simulink model "Copy_of_PDUSTM32"  (R2024b)
settings: Solver=FixedStepDiscrete  StartTime=0.0  StopTime=1  FixedStep=0.001  RelTol=1e-3  EnableMultiTasking=on
libraries: stm32blockslib x32, stm32f4xxblockslib x14, canmsglib x7, simulink x3, stm32h7xxblockslib x1
(part 1 of 3)
settings Model: STM32="{\"DigitalPortRead\":[{\"ID\":\"Copy_of_PDUSTM32:620\"},{\"ID\":\"Copy_of_PDUSTM32:1176\"},{\"ID\":\"Copy_of_PDUSTM32:1323\"}],\"SPIControllerTransfer\":[{\"ID\":\"Copy_of_PDUSTM32:1123\"},{\"ID\":\"Copy_of_PDUSTM32:1124\"},{\"ID\":\"Copy_of_PDUSTM32:1150\"},{\"ID\":\"Copy_of_PDUSTM32:1151\"},{\"ID\":\"Copy_of_PDUSTM32:1152\"},{\"ID\":\"Copy_of_PDUSTM32:1153\"},{\"ID\":\"Copy_of_PDUSTM32:1154\"},{\"ID\":\"Copy_of_PDUSTM32:1155\"},{\"ID\":\"Copy_of_PDUSTM32:1156\"},{\"ID\":\"Copy_of_PDUSTM32:1157\"},{\"ID\":\"Copy_of_PDUSTM32:709\"},{\"ID\":\"Copy_of_PDUSTM32:716\"},{\"ID\":\"Copy_of_PDUSTM32:722\"},{\"ID\":\"Copy_of_PDUSTM32:728\"},{\"ID\":\"Copy_of_PDUSTM32:1255\"},{\"ID\":\"Copy_of_PDUSTM32:1256\"},{\"ID\":\"Copy_of_PDUSTM32:1270\"},{\"ID\":\"Copy_of_PDUSTM32:1271\"},{\"ID\":\"Copy_of_PDUSTM32:1285\"},{\"ID\":\"Copy_of_PDUSTM32:1286\"},{\"ID\":\"Copy_of_PDUSTM32:1305\"},{\"ID\":\"Copy_of_PDUSTM32:1306\"},{\"ID\":\"Copy_of_PDUSTM32:1181\"},{\"ID\":\"Copy_of_PDUSTM32:1328\"},{\"ID\":\"Copy_of_PDUSTM32:1365\"},{\"ID\":\"Copy_of_PDUSTM32:1366\"},{\"ID\":\"Copy_of_PDUSTM32:1382\"},{\"ID\":\"Copy_of_PDUSTM32:1383\"},{\"ID\":\"Copy_of_PDUSTM32:1394\"},{\"ID\":\"Copy_of_PDUSTM32:1395\"},{\"ID\":\"Copy_of_PDUSTM32:1406\"},{\"ID\":\"Copy_of_PDUSTM32:1407\"}],\"AnalogInputForH7\":{\"ID\":\"Copy_of_PDUSTM32:731\"},\"DigitalPortWrite\":[{\"ID\":\"Copy_of_PDUSTM32:1095\"},{\"ID\":\"Copy_of_PDUSTM32:1094\"},{\"ID\":\"Copy_of_PDUSTM32:1093\"},{\"ID\":\"Copy_of_PDUSTM32:1092\"},{\"ID\":\"Copy_of_PDUSTM32:1091\"},{\"ID\":\"Copy_of_PDUSTM32:826\"},{\"ID\":\"Copy_of_PDUSTM32:825\"},{\"ID\":\"Copy_of_PDUSTM32:809\"},{\"ID\":\"Copy_of_PDUSTM32:921\"},{\"ID\":\"Copy_of_PDUSTM32:889\"},{\"ID\":\"Copy_of_PDUSTM32:1131\"}]}"  Creator=will  LastModifiedBy=Will
settings SolverCC: AlgebraicLoopSolver=TrustRegion
settings DataIOCC: ReturnWorkspaceOutputs=off
settings OptimizationCC: DefaultParameterBehavior=Inlined  EnhancedBackFolding=on  PassReuseOutputArgsAs=Individual arguments  ZeroExternalMemoryAtStartup=off  ZeroInternalMemoryAtStartup=off  MaxStackSize=512  OptimizeBlockOrder=speed  DifferentSizesBufferReuse=on  OptimizationCustomize=off  EfficientTunableParamExpr=on
settings DebuggingCC: ParameterTunabilityLossMsg=error  UnconnectedInputMsg=warning  UnconnectedOutputMsg=warning  UnconnectedLineMsg=warning  ArithmeticOperatorsInVariantConditions=warning
settings HardwareCC: ProdBitPerPointer=32  ProdBitPerSizeT=32  ProdBitPerPtrDiffT=32  ProdLargestAtomicInteger=Long  ProdLargestAtomicFloat=Double  ProdWordSize=32  ProdLongLongMode=on  ProdHWDeviceType=ARM Compatible->ARM Cortex-M
settings ModelReferenceCC: EnableRefExpFcnMdlSchedulingChecks=on
settings SFSimCC: MATLABDynamicMemAlloc=off  CustomCodeUndefinedFunction=UseInterfaceOnly
settings RTWCC: Description=Embedded Coder  SystemTargetFile=ert.tlc  HardwareBoard=STM32H7xx Based (Single-core)  TemplateMakefile=ert_default_tmf  CustomHeaderCode="#include \"stm32h7xx_ll_tim.h\""  CustomInitializer=LL_TIM_EnableCounter(TIM2);  Toolchain=GNU Tools for ARM Embedded Processors  GPUComputeCapability=3.5
settings CodeAppCC: ForceParamTrailComments=on  IgnoreCustomStorageClasses=off  OperatorAnnotations=on  SimulinkDataObjDesc=on  SFDataObjDesc=on  InsertBlockDesc=on
settings ERTTargetCC: TargetLangStandard=C99 (ISO)  CodeReplacementLibrary=ARM Cortex-M  ExtModeTransport=3  ExtModeStaticAlloc=on  ExtModeStaticAllocSize=2048  ExtModeMexFile=ext_xcp  ExtModeIntrfLevel=Level2 - Open

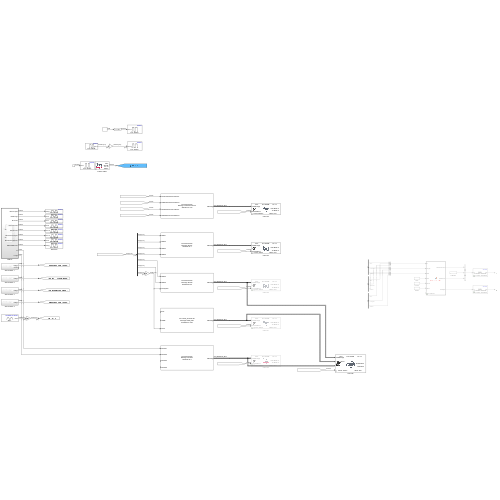
[thumbnail: Simulink's stored preview of the top-level diagram]
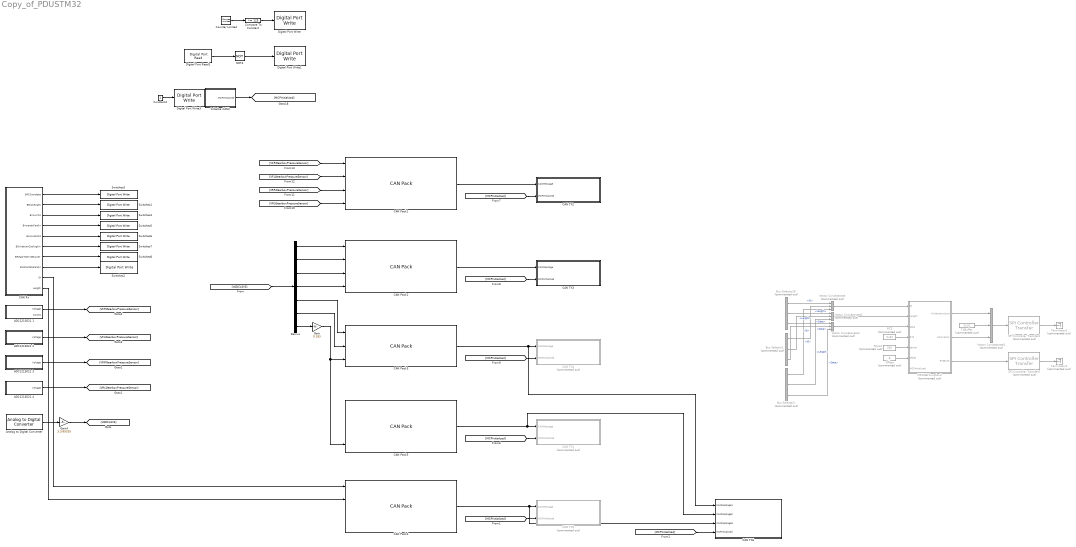
== system Copy_of_PDUSTM32 ==
  ADC121S021 1 : Subsystem
  ADC121S021 2 : Subsystem
  ADC121S021 3 : Subsystem
  ADC121S021 4 : Subsystem
  Analog to Digital Converter : stm32h7xxblockslib/Analog to Digital Converter  ADCModule=ADC1  ConversionGroup=Regular  TriggerMode=Read results only  NumberOfConversions=7  EnableBufferConv=off  BufferLength=1  OutputStatus=off  SampleTime=-1  EnableSimPort=off  hoistedMaskSrc=ECSoC/ECSimCodegen/Analog to Digital Converter
  Bus Selector1 : BusSelector  Commented=on  OutputSignals=ID,Length,Data
  Bus Selector16 : BusSelector  Commented=on  OutputSignals=ID,Length,Data
  Bus Selector2 : BusSelector  Commented=on  OutputSignals=ID,Length,Data
  CAN Pack1 : canmsglib/CAN Pack  CANdbFile=C:\Users\oxbro\Documents\STM32CustomProjects\PDUSTM32\ADCTest.dbc  MsgList=GearboxPressures  MsgName=GearboxPressures  MsgIDType=Standard (11-bit identifier)  MsgIdentifier=105  CANIDInput=off  MsgLength=8  Remote=off  ApplyMinMax=off  BusOutput=on  SignalInfo={'VFLGearboxPressureSensor','0','12','LE','unsigned','Standard','0','0.0012211','0','0','5.0004';'VFRGearboxPressureSensor','16','12','LE','unsigned','Standard','0','0.0012211','0','0','5.0004';'VRLGearboxPressureSensor','32','12','LE','unsigned','Standard','0','0.0012211','0','0','5.0004';'VRRGearboxPressureSensor','48','12','LE','unsigned','Standard','0','0.0012211','0','0','5.0004'}
      settings: LibrarySourceBlock=stmutilitieslib/CAN Pack  DataFormat=CANdb specified signals
  CAN Pack2 : canmsglib/CAN Pack  CANdbFile=C:\Users\oxbro\Documents\STM32CustomProjects\PDUSTM32\ADCTest.dbc  MsgList=ADCs1  MsgName=ADCs1  MsgIDType=Standard (11-bit identifier)  MsgIdentifier=5  CANIDInput=off  MsgLength=8  Remote=off  ApplyMinMax=off  BusOutput=on  SignalInfo={'VADC1','0','16','LE','unsigned','Standard','0','5.04e-05','0','0','3.303';'VADC2','16','16','LE','unsigned','Standard','0','5.04e-05','0','0','3.303';'VADC3','32','16','LE','unsigned','Standard','0','5.04e-05','0','0','3.303';'VADC4','48','16','LE','unsigned','Standard','0','5.04e-05','0','0','3.303'}
      settings: LibrarySourceBlock=stmutilitieslib/CAN Pack  DataFormat=CANdb specified signals
  CAN Pack3 : canmsglib/CAN Pack  CANdbFile=C:\Users\oxbro\Documents\STM32CustomProjects\PDUSTM32\ADCTest.dbc  MsgList=ADCs2  MsgName=ADCs2  MsgIDType=Standard (11-bit identifier)  MsgIdentifier=66  CANIDInput=off  MsgLength=6  Remote=off  ApplyMinMax=off  BusOutput=on  SignalInfo={'VADC5','0','16','LE','unsigned','Standard','0','5.04e-05','0','0','3.303';'VADC6','16','16','LE','unsigned','Standard','0','5.04e-05','0','0','3.303';'VLVSystem','32','16','LE','unsigned','Standard','0','0.00046327','0','0','30.3604'}
      settings: LibrarySourceBlock=stmutilitieslib/CAN Pack  DataFormat=CANdb specified signals
  CAN Pack4 : canmsglib/CAN Pack  CANdbFile=C:\Users\oxbro\Documents\STM32CustomProjects\PDUSTM32\ADCTest.dbc  MsgList=Numbers  MsgName=Numbers  MsgIDType=Standard (11-bit identifier)  MsgIdentifier=0  CANIDInput=off  MsgLength=8  Remote=off  ApplyMinMax=off  BusOutput=on  SignalInfo={'Number1','0','16','LE','signed','Standard','0','1','0','-32768','32767';'Number2','16','16','LE','signed','Standard','0','1','0','-32768','32767';'Number3','32','16','LE','signed','Standard','0','1','0','-32768','32767';'Number4','48','16','LE','signed','Standard','0','1','0','-32768','32767'}
      settings: LibrarySourceBlock=stmutilitieslib/CAN Pack  DataFormat=CANdb specified signals
  CAN Pack5 : canmsglib/CAN Pack  CANdbFile=C:\Users\Will\Desktop\OBR\Embedded\PDUSTM32\CAN3_28.06.26.dbc  MsgList=PDM_Data  MsgName=PDM_Data  MsgIDType=Standard (11-bit identifier)  MsgIdentifier=1328  CANIDInput=off  MsgLength=8  Remote=off  ApplyMinMax=off  BusOutput=on  SignalInfo={'ILVS','8','8','LE','unsigned','Standard','0','1','0','0','255';'TPDM','16','8','LE','unsigned','Standard','0','1','0','0','255';'VLVS','0','8','LE','unsigned','Standard','0','0.1216','0','0','31.008'}
      settings: LibrarySourceBlock=stmutilitieslib/CAN Pack  DataFormat=CANdb specified signals
  CAN Rx : Subsystem  TreatAsAtomicUnit=on
  CAN TX1 : Subsystem  Commented=on  mask{SPIModuleSelect=SPI1, Port_Select=GPIOB, Pin=14, SPIModule=uint32(0), Offset=6, Period=250, RTS=0x81, TXBuffer=0x31}
      mask prompts: SPIModuleSelect "SPI module:"; Port_Select "Chip select port name:"; Pin "Chip select pin number:"; SPIModule "svd:svd:SPIModulePrompt"; Offset "Offset (ms)"; Period "Period (ms)"; RTS "RTS (0x81, 0x82, 0x84)"; TXBuffer "TX Buffer (0x31, 0x41, 0x51)"
      mask TypeOptions SPIModuleSelect: SPI Controller Transfer4/SPIModuleSelect | SPI Controller Transfer5/SPIModuleSelect
      mask TypeOptions Port_Select: SPI Controller Transfer4/Port_Select | SPI Controller Transfer5/Port_Select
      mask TypeOptions Pin: SPI Controller Transfer4/Pin | SPI Controller Transfer5/Pin
      mask TypeOptions SPIModule: SPI Controller Transfer4/SPIModule | SPI Controller Transfer5/SPIModule
      mask TypeOptions Offset: Offset/Value
      mask TypeOptions Period: Period/Value
      mask TypeOptions RTS: RTS/Value
      mask TypeOptions TXBuffer: TXBuffer/Value
      mask DialogControl DescTextVar Prompt: Configure CAN TX. Please ensure RTS and TX are to the same buffer
      mask DialogControl SPIModule Prompt: SPI module
      mask Display:
      | port_label('input', 1, 'CANMessage');
      | port_label('input', 2, 'MCPInitialized');
      | 
      | % Top section: SPI config
      | text(0.2, 0.9, '' + string(get_param(gcb,'SPIModuleSelect')), HorizontalAlignment = 'center');
      | text(0.8, 0.9, 'Pin ' + string(get_param(gcb,'Pin')), HorizontalAlignment = 'center');
      | text(0.5, 0.9, 'Port ' + string(get_param(gcb,'Port_Select')), HorizontalAlignment = 'center');
      | 
      | % MCP buffer config
      | if string(get_param(gcb,'TXBuffer')) == "0x31"
      |     text(0.95, 0.35, 'TX Buffer 0', HorizontalAlignment = 'right');
      | elseif string(get_param(gcb,'TXBuffer')) == "0x41"
      |     text(0.95, 0.35, 'TX Buffer 1', HorizontalAlignment = 'right');
      | elseif string(get_param(gcb,'TXBuffer')) == "0x51"
      |     text(0.95, 0.35, 'TX Buffer 2', HorizontalAlignment = 'right');
      | else
      |     text(0.95, 0.35, 'INVALID BUFFER', HorizontalAlignment = 'right');
      | end
      | 
      | if string(get_param(gcb,'RTS')) == "0x81"
      |     text(0.95, 0.55, 'RTS Buffer 0', HorizontalAlignment = 'right');
      | elseif string(get_param(gcb,'RTS')) == "0x82"
      |     text(0.95, 0.55, 'RTS Buffer 1', HorizontalAlignment = 'right');
      | elseif string(get_param(gcb,'RTS')) == "0x84"
      |     text(0.95, 0.55, 'RTS Buffer 2', HorizontalAlignment = 'right');
      | else
      |     text(0.95, 0.55, 'INVALID BUFFER', HorizontalAlignment = 'right');
      | end
      | 
      | % text(0.95, 0.55, 'RTS: ' + string(get_param(gcb,'RTS')), HorizontalAlignment = 'right');
      | 
      | text(0.25, 0.1, 'Period: ' + string(get_param(gcb,'Period')) + 'ms', HorizontalAlignment = 'center');
      | text(0.75, 0.1, 'Offset: ' + string(get_param(gcb,'Offset')) + 'ms', HorizontalAlignment = 'center');
      | 
      | % MCP25625 logo
      | pos = get_param(gcb, 'Position');
      | blockAspect = (pos(3)-pos(1)) / (pos(4)-pos(2));
      | 
      | % fit(img, m, cx, cy): m = fraction of block the image occupies,
      | % (cx,cy) = center point in normalized 0-1 coords
      | fit = @(img,m,cx,cy) [ ...
      |     cx - m*min(1,(size(img,2)/size(img,1))/blockAspect)/2, ...
      |     cy - m*min(1,blockAspect/(size(img,2)/size(img,1)))/2, ...
      |     m*min(1,(size(img,2)/size(img,1))/blockAspect), ...
      |     m*min(1,blockAspect/(size(img,2)/size(img,1))) ];
      | 
      | ud = get_param(gcb, 'UserData');
      | 
      | image(ud.mcplogo, fit(ud.mcplogo, 0.3, 0.1, 0.5));
      | image(ud.obrlogo, fit(ud.obrlogo, 0.5, 0.5, 0.5));
  CAN TX2 : Subsystem  mask{SPIModuleSelect=SPI1, Port_Select=GPIOB, Pin=14, SPIModule=uint32(0), Offset=0, Period=5000, RTS=0x81, TXBuffer=0x31}
      mask prompts: SPIModuleSelect "SPI module:"; Port_Select "Chip select port name:"; Pin "Chip select pin number:"; SPIModule "svd:svd:SPIModulePrompt"; Offset "Offset (ms)"; Period "Period (ms)"; RTS "RTS (0x81, 0x82, 0x84)"; TXBuffer "TX Buffer (0x31, 0x41, 0x51)"
      mask TypeOptions SPIModuleSelect: SPI Controller Transfer4/SPIModuleSelect | SPI Controller Transfer5/SPIModuleSelect
      mask TypeOptions Port_Select: SPI Controller Transfer4/Port_Select | SPI Controller Transfer5/Port_Select
      mask TypeOptions Pin: SPI Controller Transfer4/Pin | SPI Controller Transfer5/Pin
      mask TypeOptions SPIModule: SPI Controller Transfer4/SPIModule | SPI Controller Transfer5/SPIModule
      mask TypeOptions Offset: Offset/Value
      mask TypeOptions Period: Period/Value
      mask TypeOptions RTS: RTS/Value
      mask TypeOptions TXBuffer: TXBuffer/Value
      mask DialogControl DescTextVar Prompt: Configure CAN TX. Please ensure RTS and TX are to the same buffer
      mask DialogControl SPIModule Prompt: SPI module
      mask Display:
      | port_label('input', 1, 'CANMessage');
      | port_label('input', 2, 'MCPInitialized');
      | 
      | % Top section: SPI config
      | text(0.2, 0.9, '' + string(get_param(gcb,'SPIModuleSelect')), HorizontalAlignment = 'center');
      | text(0.8, 0.9, 'Pin ' + string(get_param(gcb,'Pin')), HorizontalAlignment = 'center');
      | text(0.5, 0.9, 'Port ' + string(get_param(gcb,'Port_Select')), HorizontalAlignment = 'center');
      | 
      | % MCP buffer config
      | if string(get_param(gcb,'TXBuffer')) == "0x31"
      |     text(0.95, 0.35, 'TX Buffer 0', HorizontalAlignment = 'right');
      | elseif string(get_param(gcb,'TXBuffer')) == "0x41"
      |     text(0.95, 0.35, 'TX Buffer 1', HorizontalAlignment = 'right');
      | elseif string(get_param(gcb,'TXBuffer')) == "0x51"
      |     text(0.95, 0.35, 'TX Buffer 2', HorizontalAlignment = 'right');
      | else
      |     text(0.95, 0.35, 'INVALID BUFFER', HorizontalAlignment = 'right');
      | end
      | 
      | if string(get_param(gcb,'RTS')) == "0x81"
      |     text(0.95, 0.55, 'RTS Buffer 0', HorizontalAlignment = 'right');
      | elseif string(get_param(gcb,'RTS')) == "0x82"
      |     text(0.95, 0.55, 'RTS Buffer 1', HorizontalAlignment = 'right');
      | elseif string(get_param(gcb,'RTS')) == "0x84"
      |     text(0.95, 0.55, 'RTS Buffer 2', HorizontalAlignment = 'right');
      | else
      |     text(0.95, 0.55, 'INVALID BUFFER', HorizontalAlignment = 'right');
      | end
      | 
      | % text(0.95, 0.55, 'RTS: ' + string(get_param(gcb,'RTS')), HorizontalAlignment = 'right');
      | 
      | text(0.25, 0.1, 'Period: ' + string(get_param(gcb,'Period')) + 'ms', HorizontalAlignment = 'center');
      | text(0.75, 0.1, 'Offset: ' + string(get_param(gcb,'Offset')) + 'ms', HorizontalAlignment = 'center');
      | 
      | % MCP25625 logo
      | pos = get_param(gcb, 'Position');
      | blockAspect = (pos(3)-pos(1)) / (pos(4)-pos(2));
      | 
      | % fit(img, m, cx, cy): m = fraction of block the image occupies,
      | % (cx,cy) = center point in normalized 0-1 coords
      | fit = @(img,m,cx,cy) [ ...
      |     cx - m*min(1,(size(img,2)/size(img,1))/blockAspect)/2, ...
      |     cy - m*min(1,blockAspect/(size(img,2)/size(img,1)))/2, ...
      |     m*min(1,(size(img,2)/size(img,1))/blockAspect), ...
      |     m*min(1,blockAspect/(size(img,2)/size(img,1))) ];
      | 
      | ud = get_param(gcb, 'UserData');
      | 
      | image(ud.mcplogo, fit(ud.mcplogo, 0.3, 0.1, 0.5));
      | image(ud.obrlogo, fit(ud.obrlogo, 0.5, 0.5, 0.5));
  CAN TX3 : Subsystem  mask{SPIModuleSelect=SPI1, Port_Select=GPIOB, Pin=14, SPIModule=uint32(0), Offset=2, Period=250, RTS=0x81, TXBuffer=0x31}
      mask prompts: SPIModuleSelect "SPI module:"; Port_Select "Chip select port name:"; Pin "Chip select pin number:"; SPIModule "svd:svd:SPIModulePrompt"; Offset "Offset (ms)"; Period "Period (ms)"; RTS "RTS (0x81, 0x82, 0x84)"; TXBuffer "TX Buffer (0x31, 0x41, 0x51)"
      mask TypeOptions SPIModuleSelect: SPI Controller Transfer4/SPIModuleSelect | SPI Controller Transfer5/SPIModuleSelect
      mask TypeOptions Port_Select: SPI Controller Transfer4/Port_Select | SPI Controller Transfer5/Port_Select
      mask TypeOptions Pin: SPI Controller Transfer4/Pin | SPI Controller Transfer5/Pin
      mask TypeOptions SPIModule: SPI Controller Transfer4/SPIModule | SPI Controller Transfer5/SPIModule
      mask TypeOptions Offset: Offset/Value
      mask TypeOptions Period: Period/Value
      mask TypeOptions RTS: RTS/Value
      mask TypeOptions TXBuffer: TXBuffer/Value
      mask DialogControl DescTextVar Prompt: Configure CAN TX. Please ensure RTS and TX are to the same buffer
      mask DialogControl SPIModule Prompt: SPI module
      mask Display:
      | port_label('input', 1, 'CANMessage');
      | port_label('input', 2, 'MCPInitialized');
      | 
      | % Top section: SPI config
      | text(0.2, 0.9, '' + string(get_param(gcb,'SPIModuleSelect')), HorizontalAlignment = 'center');
      | text(0.8, 0.9, 'Pin ' + string(get_param(gcb,'Pin')), HorizontalAlignment = 'center');
      | text(0.5, 0.9, 'Port ' + string(get_param(gcb,'Port_Select')), HorizontalAlignment = 'center');
      | 
      | % MCP buffer config
      | if string(get_param(gcb,'TXBuffer')) == "0x31"
      |     text(0.95, 0.35, 'TX Buffer 0', HorizontalAlignment = 'right');
      | elseif string(get_param(gcb,'TXBuffer')) == "0x41"
      |     text(0.95, 0.35, 'TX Buffer 1', HorizontalAlignment = 'right');
      | elseif string(get_param(gcb,'TXBuffer')) == "0x51"
      |     text(0.95, 0.35, 'TX Buffer 2', HorizontalAlignment = 'right');
      | else
      |     text(0.95, 0.35, 'INVALID BUFFER', HorizontalAlignment = 'right');
      | end
      | 
      | if string(get_param(gcb,'RTS')) == "0x81"
      |     text(0.95, 0.55, 'RTS Buffer 0', HorizontalAlignment = 'right');
      | elseif string(get_param(gcb,'RTS')) == "0x82"
      |     text(0.95, 0.55, 'RTS Buffer 1', HorizontalAlignment = 'right');
      | elseif string(get_param(gcb,'RTS')) == "0x84"
      |     text(0.95, 0.55, 'RTS Buffer 2', HorizontalAlignment = 'right');
      | else
      |     text(0.95, 0.55, 'INVALID BUFFER', HorizontalAlignment = 'right');
      | end
      | 
      | % text(0.95, 0.55, 'RTS: ' + string(get_param(gcb,'RTS')), HorizontalAlignment = 'right');
      | 
      | text(0.25, 0.1, 'Period: ' + string(get_param(gcb,'Period')) + 'ms', HorizontalAlignment = 'center');
      | text(0.75, 0.1, 'Offset: ' + string(get_param(gcb,'Offset')) + 'ms', HorizontalAlignment = 'center');
      | 
      | % MCP25625 logo
      | pos = get_param(gcb, 'Position');
      | blockAspect = (pos(3)-pos(1)) / (pos(4)-pos(2));
      | 
      | % fit(img, m, cx, cy): m = fraction of block the image occupies,
      | % (cx,cy) = center point in normalized 0-1 coords
      | fit = @(img,m,cx,cy) [ ...
      |     cx - m*min(1,(size(img,2)/size(img,1))/blockAspect)/2, ...
      |     cy - m*min(1,blockAspect/(size(img,2)/size(img,1)))/2, ...
      |     m*min(1,(size(img,2)/size(img,1))/blockAspect), ...
      |     m*min(1,blockAspect/(size(img,2)/size(img,1))) ];
      | 
      | ud = get_param(gcb, 'UserData');
      | 
      | image(ud.mcplogo, fit(ud.mcplogo, 0.3, 0.1, 0.5));
      | image(ud.obrlogo, fit(ud.obrlogo, 0.5, 0.5, 0.5));
  CAN TX4 : Subsystem  Commented=on  mask{SPIModuleSelect=SPI1, Port_Select=GPIOB, Pin=14, SPIModule=uint32(0), Offset=4, Period=250, RTS=0x81, TXBuffer=0x31}
      mask prompts: SPIModuleSelect "SPI module:"; Port_Select "Chip select port name:"; Pin "Chip select pin number:"; SPIModule "svd:svd:SPIModulePrompt"; Offset "Offset (ms)"; Period "Period (ms)"; RTS "RTS (0x81, 0x82, 0x84)"; TXBuffer "TX Buffer (0x31, 0x41, 0x51)"
      mask TypeOptions SPIModuleSelect: SPI Controller Transfer4/SPIModuleSelect | SPI Controller Transfer5/SPIModuleSelect
      mask TypeOptions Port_Select: SPI Controller Transfer4/Port_Select | SPI Controller Transfer5/Port_Select
      mask TypeOptions Pin: SPI Controller Transfer4/Pin | SPI Controller Transfer5/Pin
      mask TypeOptions SPIModule: SPI Controller Transfer4/SPIModule | SPI Controller Transfer5/SPIModule
      mask TypeOptions Offset: Offset/Value
      mask TypeOptions Period: Period/Value
      mask TypeOptions RTS: RTS/Value
      mask TypeOptions TXBuffer: TXBuffer/Value
      mask DialogControl DescTextVar Prompt: Configure CAN TX. Please ensure RTS and TX are to the same buffer
      mask DialogControl SPIModule Prompt: SPI module
      mask Display:
      | port_label('input', 1, 'CANMessage');
      | port_label('input', 2, 'MCPInitialized');
      | 
      | % Top section: SPI config
      | text(0.2, 0.9, '' + string(get_param(gcb,'SPIModuleSelect')), HorizontalAlignment = 'center');
      | text(0.8, 0.9, 'Pin ' + string(get_param(gcb,'Pin')), HorizontalAlignment = 'center');
      | text(0.5, 0.9, 'Port ' + string(get_param(gcb,'Port_Select')), HorizontalAlignment = 'center');
      | 
      | % MCP buffer config
      | if string(get_param(gcb,'TXBuffer')) == "0x31"
      |     text(0.95, 0.35, 'TX Buffer 0', HorizontalAlignment = 'right');
      | elseif string(get_param(gcb,'TXBuffer')) == "0x41"
      |     text(0.95, 0.35, 'TX Buffer 1', HorizontalAlignment = 'right');
      | elseif string(get_param(gcb,'TXBuffer')) == "0x51"
      |     text(0.95, 0.35, 'TX Buffer 2', HorizontalAlignment = 'right');
      | else
      |     text(0.95, 0.35, 'INVALID BUFFER', HorizontalAlignment = 'right');
      | end
      | 
      | if string(get_param(gcb,'RTS')) == "0x81"
      |     text(0.95, 0.55, 'RTS Buffer 0', HorizontalAlignment = 'right');
      | elseif string(get_param(gcb,'RTS')) == "0x82"
      |     text(0.95, 0.55, 'RTS Buffer 1', HorizontalAlignment = 'right');
      | elseif string(get_param(gcb,'RTS')) == "0x84"
      |     text(0.95, 0.55, 'RTS Buffer 2', HorizontalAlignment = 'right');
      | else
      |     text(0.95, 0.55, 'INVALID BUFFER', HorizontalAlignment = 'right');
      | end
      | 
      | % text(0.95, 0.55, 'RTS: ' + string(get_param(gcb,'RTS')), HorizontalAlignment = 'right');
      | 
      | text(0.25, 0.1, 'Period: ' + string(get_param(gcb,'Period')) + 'ms', HorizontalAlignment = 'center');
      | text(0.75, 0.1, 'Offset: ' + string(get_param(gcb,'Offset')) + 'ms', HorizontalAlignment = 'center');
      | 
      | % MCP25625 logo
      | pos = get_param(gcb, 'Position');
      | blockAspect = (pos(3)-pos(1)) / (pos(4)-pos(2));
      | 
      | % fit(img, m, cx, cy): m = fraction of block the image occupies,
      | % (cx,cy) = center point in normalized 0-1 coords
      | fit = @(img,m,cx,cy) [ ...
      |     cx - m*min(1,(size(img,2)/size(img,1))/blockAspect)/2, ...
      |     cy - m*min(1,blockAspect/(size(img,2)/size(img,1)))/2, ...
      |     m*min(1,(size(img,2)/size(img,1))/blockAspect), ...
      |     m*min(1,blockAspect/(size(img,2)/size(img,1))) ];
      | 
      | ud = get_param(gcb, 'UserData');
      | 
      | image(ud.mcplogo, fit(ud.mcplogo, 0.3, 0.1, 0.5));
      | image(ud.obrlogo, fit(ud.obrlogo, 0.5, 0.5, 0.5));
  CAN TX5 : Subsystem  Commented=on  mask{SPIModuleSelect=SPI1, Port_Select=GPIOB, Pin=14, SPIModule=uint32(0), Offset=8, Period=250, RTS=0x81, TXBuffer=0x31}
      mask prompts: SPIModuleSelect "SPI module:"; Port_Select "Chip select port name:"; Pin "Chip select pin number:"; SPIModule "svd:svd:SPIModulePrompt"; Offset "Offset (ms)"; Period "Period (ms)"; RTS "RTS (0x81, 0x82, 0x84)"; TXBuffer "TX Buffer (0x31, 0x41, 0x51)"
      mask TypeOptions SPIModuleSelect: SPI Controller Transfer4/SPIModuleSelect | SPI Controller Transfer5/SPIModuleSelect
      mask TypeOptions Port_Select: SPI Controller Transfer4/Port_Select | SPI Controller Transfer5/Port_Select
      mask TypeOptions Pin: SPI Controller Transfer4/Pin | SPI Controller Transfer5/Pin
      mask TypeOptions SPIModule: SPI Controller Transfer4/SPIModule | SPI Controller Transfer5/SPIModule
      mask TypeOptions Offset: Offset/Value
      mask TypeOptions Period: Period/Value
      mask TypeOptions RTS: RTS/Value
      mask TypeOptions TXBuffer: TXBuffer/Value
      mask DialogControl DescTextVar Prompt: Configure CAN TX. Please ensure RTS and TX are to the same buffer
      mask DialogControl SPIModule Prompt: SPI module
      mask Display:
      | port_label('input', 1, 'CANMessage');
      | port_label('input', 2, 'MCPInitialized');
      | 
      | % Top section: SPI config
      | text(0.2, 0.9, '' + string(get_param(gcb,'SPIModuleSelect')), HorizontalAlignment = 'center');
      | text(0.8, 0.9, 'Pin ' + string(get_param(gcb,'Pin')), HorizontalAlignment = 'center');
      | text(0.5, 0.9, 'Port ' + string(get_param(gcb,'Port_Select')), HorizontalAlignment = 'center');
      | 
      | % MCP buffer config
      | if string(get_param(gcb,'TXBuffer')) == "0x31"
      |     text(0.95, 0.35, 'TX Buffer 0', HorizontalAlignment = 'right');
      | elseif string(get_param(gcb,'TXBuffer')) == "0x41"
      |     text(0.95, 0.35, 'TX Buffer 1', HorizontalAlignment = 'right');
      | elseif string(get_param(gcb,'TXBuffer')) == "0x51"
      |     text(0.95, 0.35, 'TX Buffer 2', HorizontalAlignment = 'right');
      | else
      |     text(0.95, 0.35, 'INVALID BUFFER', HorizontalAlignment = 'right');
      | end
      | 
      | if string(get_param(gcb,'RTS')) == "0x81"
      |     text(0.95, 0.55, 'RTS Buffer 0', HorizontalAlignment = 'right');
      | elseif string(get_param(gcb,'RTS')) == "0x82"
      |     text(0.95, 0.55, 'RTS Buffer 1', HorizontalAlignment = 'right');
      | elseif string(get_param(gcb,'RTS')) == "0x84"
      |     text(0.95, 0.55, 'RTS Buffer 2', HorizontalAlignment = 'right');
      | else
      |     text(0.95, 0.55, 'INVALID BUFFER', HorizontalAlignment = 'right');
      | end
      | 
      | % text(0.95, 0.55, 'RTS: ' + string(get_param(gcb,'RTS')), HorizontalAlignment = 'right');
      | 
      | text(0.25, 0.1, 'Period: ' + string(get_param(gcb,'Period')) + 'ms', HorizontalAlignment = 'center');
      | text(0.75, 0.1, 'Offset: ' + string(get_param(gcb,'Offset')) + 'ms', HorizontalAlignment = 'center');
      | 
      | % MCP25625 logo
      | pos = get_param(gcb, 'Position');
      | blockAspect = (pos(3)-pos(1)) / (pos(4)-pos(2));
      | 
      | % fit(img, m, cx, cy): m = fraction of block the image occupies,
      | % (cx,cy) = center point in normalized 0-1 coords
      | fit = @(img,m,cx,cy) [ ...
      |     cx - m*min(1,(size(img,2)/size(img,1))/blockAspect)/2, ...
      |     cy - m*min(1,blockAspect/(size(img,2)/size(img,1)))/2, ...
      |     m*min(1,(size(img,2)/size(img,1))/blockAspect), ...
      |     m*min(1,blockAspect/(size(img,2)/size(img,1))) ];
      | 
      | ud = get_param(gcb, 'UserData');
      | 
      | image(ud.mcplogo, fit(ud.mcplogo, 0.3, 0.1, 0.5));
      | image(ud.obrlogo, fit(ud.obrlogo, 0.5, 0.5, 0.5));
  CAN TX6 : Subsystem  mask{SPIModuleSelect=SPI1, Port_Select=GPIOB, Pin=14, SPIModule=uint32(0), Offset=8, Period=250, RTS=0x81, TXBuffer=0x31}
      mask prompts: SPIModuleSelect "SPI module:"; Port_Select "Chip select port name:"; Pin "Chip select pin number:"; SPIModule "svd:svd:SPIModulePrompt"; Offset "Offset (ms)"; Period "Period (ms)"; RTS "RTS (0x81, 0x82, 0x84)"; TXBuffer "TX Buffer (0x31, 0x41, 0x51)"
      mask TypeOptions SPIModuleSelect: SPI Controller Transfer4/SPIModuleSelect | SPI Controller Transfer5/SPIModuleSelect
      mask TypeOptions Port_Select: SPI Controller Transfer4/Port_Select | SPI Controller Transfer5/Port_Select
      mask TypeOptions Pin: SPI Controller Transfer4/Pin | SPI Controller Transfer5/Pin
      mask TypeOptions SPIModule: SPI Controller Transfer4/SPIModule | SPI Controller Transfer5/SPIModule
      mask TypeOptions Offset: Offset/Value
      mask TypeOptions Period: Period/Value
      mask TypeOptions RTS: RTS/Value
      mask TypeOptions TXBuffer: TXBuffer/Value
      mask DialogControl DescTextVar Prompt: Configure CAN TX. Please ensure RTS and TX are to the same buffer
      mask DialogControl SPIModule Prompt: SPI module
      mask Display:
      | port_label('input', 1, 'CANMessage');
      | port_label('input', 2, 'MCPInitialized');
      | 
      | % Top section: SPI config
      | text(0.2, 0.9, '' + string(get_param(gcb,'SPIModuleSelect')), HorizontalAlignment = 'center');
      | text(0.8, 0.9, 'Pin ' + string(get_param(gcb,'Pin')), HorizontalAlignment = 'center');
      | text(0.5, 0.9, 'Port ' + string(get_param(gcb,'Port_Select')), HorizontalAlignment = 'center');
      | 
      | % MCP buffer config
      | if string(get_param(gcb,'TXBuffer')) == "0x31"
      |     text(0.95, 0.35, 'TX Buffer 0', HorizontalAlignment = 'right');
      | elseif string(get_param(gcb,'TXBuffer')) == "0x41"
      |     text(0.95, 0.35, 'TX Buffer 1', HorizontalAlignment = 'right');
      | elseif string(get_param(gcb,'TXBuffer')) == "0x51"
      |     text(0.95, 0.35, 'TX Buffer 2', HorizontalAlignment = 'right');
      | else
      |     text(0.95, 0.35, 'INVALID BUFFER', HorizontalAlignment = 'right');
      | end
      | 
      | if string(get_param(gcb,'RTS')) == "0x81"
      |     text(0.95, 0.55, 'RTS Buffer 0', HorizontalAlignment = 'right');
      | elseif string(get_param(gcb,'RTS')) == "0x82"
      |     text(0.95, 0.55, 'RTS Buffer 1', HorizontalAlignment = 'right');
      | elseif string(get_param(gcb,'RTS')) == "0x84"
      |     text(0.95, 0.55, 'RTS Buffer 2', HorizontalAlignment = 'right');
      | else
      |     text(0.95, 0.55, 'INVALID BUFFER', HorizontalAlignment = 'right');
      | end
      | 
      | % text(0.95, 0.55, 'RTS: ' + string(get_param(gcb,'RTS')), HorizontalAlignment = 'right');
      | 
      | text(0.25, 0.1, 'Period: ' + string(get_param(gcb,'Period')) + 'ms', HorizontalAlignment = 'center');
      | text(0.75, 0.1, 'Offset: ' + string(get_param(gcb,'Offset')) + 'ms', HorizontalAlignment = 'center');
      | 
      | % MCP25625 logo
      | pos = get_param(gcb, 'Position');
      | blockAspect = (pos(3)-pos(1)) / (pos(4)-pos(2));
      | 
      | % fit(img, m, cx, cy): m = fraction of block the image occupies,
      | % (cx,cy) = center point in normalized 0-1 coords
      | fit = @(img,m,cx,cy) [ ...
      |     cx - m*min(1,(size(img,2)/size(img,1))/blockAspect)/2, ...
      |     cy - m*min(1,blockAspect/(size(img,2)/size(img,1)))/2, ...
      |     m*min(1,(size(img,2)/size(img,1))/blockAspect), ...
      |     m*min(1,blockAspect/(size(img,2)/size(img,1))) ];
      | 
      | ud = get_param(gcb, 'UserData');
      | 
      | image(ud.mcplogo, fit(ud.mcplogo, 0.3, 0.1, 0.5));
      | image(ud.obrlogo, fit(ud.obrlogo, 0.5, 0.5, 0.5));
  Compare To Constant : simulink/Logic and Bit Operations/Compare To Constant  relop=>=  const=125  OutDataTypeStr=boolean
  Constant4 : Constant  OutDataTypeStr=boolean
  Counter Limited : simulink/Sources/Counter Limited  uplimit=250  tsamp=-1
  Demux : Demux  Outputs=7
  Digital Port Read1 : stm32f4xxblockslib/Digital Port Read  PortName=GPIOB  PinNumber=2  ReadOperation=on  IOAsArray=off  SampleTime=-1  EnableSimPort=off  hoistedMaskSrc=ECSoC/ECSimCodegen/Digital Port Read
      settings: LibrarySourceBlock=stm32f2xxblockslib/Digital Port Read
  Digital Port Write : stm32f4xxblockslib/Digital Port Write  PortName=GPIOC  PinNumber=11  ReadOperation=off  IOAsArray=off  EnableSimPort=off  hoistedMaskSrc=ECSoC/ECSimCodegen/Digital Port Write
      settings: LibrarySourceBlock=stm32h7xxblockslib/Digital Port Write
  Digital Port Write1 : stm32f4xxblockslib/Digital Port Write  PortName=GPIOC  PinNumber=12  ReadOperation=off  IOAsArray=off  EnableSimPort=off  hoistedMaskSrc=ECSoC/ECSimCodegen/Digital Port Write
      settings: LibrarySourceBlock=stm32h7xxblockslib/Digital Port Write
  Digital Port Write3 : stm32f4xxblockslib/Digital Port Write  PortName=GPIOA  PinNumber=1  ReadOperation=off  IOAsArray=off  EnableSimPort=off  hoistedMaskSrc=ECSoC/ECSimCodegen/Digital Port Write
      settings: LibrarySourceBlock=stm32h7xxblockslib/Digital Port Write
  Gain : Gain  Gain=9.183
  Gain4 : Gain  Gain=3.3/65535  OutDataTypeStr=single
  Initialize CAN3 : Subsystem  mask{SPIModuleSelect=SPI1, Port_Select=GPIOB, Pin=14, BaudConfig=0xC0}
      mask prompts: SPIModuleSelect "SPI Module"; Port_Select "CS Port"; Pin "CS Pin"; BaudConfig "Baud Byte (0xC0 = 1mb/s, 0xC1 = 500kb/s)"
      mask TypeOptions SPIModuleSelect: MCPInit/SPI Controller Transfer/SPIModuleSelect | MCPInit/SPI Controller Transfer1/SPIModuleSelect | MCPInit/SPI Controller Transfer2/SPIModuleSelect | MCPInit/SPI Controller Transfer3/SPIModuleSelect | MCPInit/SPI Controller Transfer4/SPIModuleSelect | MCPInit/SPI Controller Transfer5/SPIModuleSelect | MCPInit/SPI Controller Transfer6/SPIModuleSelect | MCPInit/SPI Controller Transfer7/SPIModuleSelect
      mask TypeOptions Port_Select: MCPInit/SPI Controller Transfer/Port_Select | MCPInit/SPI Controller Transfer1/Port_Select | MCPInit/SPI Controller Transfer2/Port_Select | MCPInit/SPI Controller Transfer3/Port_Select | MCPInit/SPI Controller Transfer4/Port_Select | MCPInit/SPI Controller Transfer5/Port_Select | MCPInit/SPI Controller Transfer6/Port_Select | MCPInit/SPI Controller Transfer7/Port_Select
      mask TypeOptions Pin: MCPInit/SPI Controller Transfer/Pin | MCPInit/SPI Controller Transfer1/Pin | MCPInit/SPI Controller Transfer2/Pin | MCPInit/SPI Controller Transfer3/Pin | MCPInit/SPI Controller Transfer4/Pin | MCPInit/SPI Controller Transfer5/Pin | MCPInit/SPI Controller Transfer6/Pin | MCPInit/SPI Controller Transfer7/Pin
      mask TypeOptions BaudConfig: MCPInit/BaudConfig/Value
      mask DialogControl DescTextVar Prompt: Your current setup uses a Baud Rate Prescaler of 0 (CNF1 = 0xC0), which divides the 20 MHz clock to yield 10 Time Quanta per bit at 1000 kb/s.  By changing the BRP field bits from 0 to 1 (CNF1 = 0xC1), you double the length of each Time Quantum, effectively cutting the bus speed in half to 500 kb/s while leaving your sample point (70%) and bit timings identical.
      mask Display:
      | text(0.95, 0.8, '' + string(get_param(gcb,'SPIModuleSelect')), HorizontalAlignment = 'right');
      | text(0.95, 0.6, '' + string(get_param(gcb,'Port_Select')), HorizontalAlignment = 'right');
      | text(0.95, 0.4, 'Pin ' + string(get_param(gcb,'Pin')), HorizontalAlignment = 'right');
      | 
      | if string(get_param(gcb,'BaudConfig')) == "0xC0"
      |     text(0.95, 0.2, '1Mbit/s', HorizontalAlignment = 'right');
      | elseif string(get_param(gcb,'BaudConfig')) == "0xC1"
      |     text(0.95, 0.2, '500kbit/s', HorizontalAlignment = 'right');
      | else
      |     text(0.95, 0.2, 'INVALID BAUD', HorizontalAlignment = 'right');
      | end
      | 
      | 
      | % OBR Logo
      | pos = get_param(gcb, 'Position');
      | blockAspect = (pos(3)-pos(1)) / (pos(4)-pos(2));
      | 
      | % fit(img, m, cx, cy): m = fraction of block the image occupies,
      | % (cx,cy) = center point in normalized 0-1 coords
      | fit = @(img,m,cx,cy) [ ...
      |     cx - m*min(1,(size(img,2)/size(img,1))/blockAspect)/2, ...
      |     cy - m*min(1,blockAspect/(size(img,2)/size(img,1)))/2, ...
      |     m*min(1,(size(img,2)/size(img,1))/blockAspect), ...
      |     m*min(1,blockAspect/(size(img,2)/size(img,1))) ];
      | 
      | ud = get_param(gcb, 'UserData');
      | 
      | image(ud.obrlogo, fit(ud.obrlogo, 0.75, 0.3, 0.5));
  MATLAB Function2 : MATLAB Function  Commented=on  TreatAsAtomicUnit=on
  NOT4 : Logic  Operator=NOT  IconShape=distinctive  AllPortsSameDT=off  OutDataTypeStr=boolean
  Offset : Constant  Commented=on  Value=8  OutDataTypeStr=uint16  SampleTime=-1
  Period : Constant  Commented=on  Value=250  OutDataTypeStr=uint16  SampleTime=-1
  RTS : Constant  Commented=on  Value=0x81  OutDataTypeStr=uint8  SampleTime=-1
  SPI Controller Transfer4 : stm32blockslib/SPI Controller Transfer  Priority=1  Commented=on  SPIModuleSelect=SPI1  ClockPolarity=Low  ClockPhase=1 Edge  SPIModule=SPIModule  Mode=Master  BusSpeed=uint32(1000000)  FirstBitToTransfer=Most significant bit (MSB)  ClockMode=0  BlockFunction=Transfer  EnableRegisterAddress=off  RegisterAddress=0  OutputDataType=uint8  OutputDataLength=1  OutputStatus=off  BlockingMode=off  Timeout=0.01  DataBits=8  UseCustomSSPin=Explicit GPIO calls  ActiveLowSSPin=Active low  Port_Select=GPIOB  Pin=14
      settings: LibrarySourceBlock=stm32h7xxblockslib/SPI Controller Transfer
  SPI Controller Transfer5 : stm32blockslib/SPI Controller Transfer  Priority=2  Commented=on  SPIModuleSelect=SPI1  ClockPolarity=Low  ClockPhase=1 Edge  SPIModule=SPIModule  Mode=Master  BusSpeed=uint32(1000000)  FirstBitToTransfer=Most significant bit (MSB)  ClockMode=0  BlockFunction=Transfer  EnableRegisterAddress=off  RegisterAddress=0  OutputDataType=uint8  OutputDataLength=1  OutputStatus=off  BlockingMode=off  Timeout=0.01  DataBits=8  UseCustomSSPin=Explicit GPIO calls  ActiveLowSSPin=Active low  Port_Select=GPIOB  Pin=14
      settings: LibrarySourceBlock=stm32h7xxblockslib/SPI Controller Transfer
  Switches1 : stm32f4xxblockslib/Digital Port Write  PortName=GPIOB  PinNumber=5  ReadOperation=off  IOAsArray=off  EnableSimPort=off  hoistedMaskSrc=ECSoC/ECSimCodegen/Digital Port Write
      settings: LibrarySourceBlock=stm32h7xxblockslib/Digital Port Write
  Switches2 : stm32f4xxblockslib/Digital Port Write  PortName=GPIOC  PinNumber=[2]  ReadOperation=off  IOAsArray=on  EnableSimPort=off  hoistedMaskSrc=ECSoC/ECSimCodegen/Digital Port Write
      settings: LibrarySourceBlock=stm32h7xxblockslib/Digital Port Write
  Switches3 : stm32f4xxblockslib/Digital Port Write  PortName=GPIOA  PinNumber=[12]  ReadOperation=off  IOAsArray=on  EnableSimPort=off  hoistedMaskSrc=ECSoC/ECSimCodegen/Digital Port Write
      settings: LibrarySourceBlock=stm32h7xxblockslib/Digital Port Write
  Switches4 : stm32f4xxblockslib/Digital Port Write  PortName=GPIOB  PinNumber=7  ReadOperation=off  IOAsArray=off  EnableSimPort=off  hoistedMaskSrc=ECSoC/ECSimCodegen/Digital Port Write
      settings: LibrarySourceBlock=stm32h7xxblockslib/Digital Port Write
  Switches5 : stm32f4xxblockslib/Digital Port Write  PortName=GPIOB  PinNumber=9  ReadOperation=off  IOAsArray=off  EnableSimPort=off  hoistedMaskSrc=ECSoC/ECSimCodegen/Digital Port Write
      settings: LibrarySourceBlock=stm32h7xxblockslib/Digital Port Write
  Switches6 : stm32f4xxblockslib/Digital Port Write  PortName=GPIOB  PinNumber=12  ReadOperation=off  IOAsArray=off  EnableSimPort=off  hoistedMaskSrc=ECSoC/ECSimCodegen/Digital Port Write
      settings: LibrarySourceBlock=stm32h7xxblockslib/Digital Port Write
  Switches7 : stm32f4xxblockslib/Digital Port Write  PortName=GPIOB  PinNumber=13  ReadOperation=off  IOAsArray=off  EnableSimPort=off  hoistedMaskSrc=ECSoC/ECSimCodegen/Digital Port Write
      settings: LibrarySourceBlock=stm32h7xxblockslib/Digital Port Write
  Switches8 : stm32f4xxblockslib/Digital Port Write  PortName=GPIOB  PinNumber=4  ReadOperation=off  IOAsArray=off  EnableSimPort=off  hoistedMaskSrc=ECSoC/ECSimCodegen/Digital Port Write
      settings: LibrarySourceBlock=stm32h7xxblockslib/Digital Port Write
  TXBuffer : Constant  Commented=on  Value=0x31  OutDataTypeStr=uint8  SampleTime=-1
  Terminator1 : Terminator  Commented=on
  Terminator2 : Terminator  Commented=on
  Vector Concatenate{,1..3} (4 alike) : Concatenate  Commented=on  NumInputs=3
  wires:
  NOT4/1 -> Digital Port Write1/1
  Digital Port Read1/1 -> NOT4/1
  Analog to Digital Converter/1 -> Gain4/1
  Gain4/1 -> [VADCs3V3]
  [VADCs3V3] -> Demux/1
  ADC121S021 1/1(Voltage) -> [VFRGearboxPressureSensor]
  ADC121S021 2/1(Voltage) -> [VFLGearboxPressureSensor]
  ADC121S021 3/1(Voltage) -> [VRRGearboxPressureSensor]
  ADC121S021 4/1(Voltage) -> [VRLGearboxPressureSensor]
  CAN Rx/1(BPCComplete) -> Switches3/1
  CAN Rx/2(BBrakeLight) -> Switches1/1
  CAN Rx/8(BMotorRBHFanOn) -> Switches2/1
  Counter Limited/1 -> Compare To Constant/1
  Compare To Constant/1 -> Digital Port Write/1
  Demux/7 -> Gain/1
  Demux/6 -> CAN Pack3/2
  Demux/5 -> CAN Pack3/1
  Demux/4 -> CAN Pack2/4
  Demux/3 -> CAN Pack2/3
  Demux/2 -> CAN Pack2/2
  Demux/1 -> CAN Pack2/1
  Gain/1 -> CAN Pack3/3, CAN Pack5/3
  CAN Rx/3(BInvLVOn) -> Switches4/1
  CAN Rx/4(BInverterFanOn) -> Switches5/1
  CAN Rx/5(BAccuFanOn) -> Switches6/1
  CAN Rx/6(BDrivetrainCoolingOn) -> Switches7/1
  CAN Rx/7(BReadyToDriveBuzzer) -> Switches8/1
  [MCPInitialized] -> CAN TX1/2(MCPInitialized)
  Initialize CAN3/1(MCPInitialized) -> [MCPInitialized]
  Constant4/1 -> Digital Port Write3/1
  CAN Pack5/1 -> CAN TX6/2(CANMessage2), CAN TX1/1(CANMessage)
  CAN Pack1/1 -> CAN TX2/1(CANMessage)
  [MCPInitialized] -> CAN TX2/2(MCPInitialized)
  [MCPInitialized] -> CAN TX3/2(MCPInitialized)
  CAN Pack2/1 -> CAN TX3/1(CANMessage)
  [MCPInitialized] -> CAN TX4/2(MCPInitialized)
  CAN Pack3/1 -> CAN TX6/1(CANMessage1), CAN TX4/1(CANMessage)
  [VRLGearboxPressureSensor] -> CAN Pack1/4
  [VRRGearboxPressureSensor] -> CAN Pack1/3
  [VFLGearboxPressureSensor] -> CAN Pack1/2
  [VFRGearboxPressureSensor] -> CAN Pack1/1
  CAN Pack4/1 -> CAN TX6/3(CANMessage3), CAN TX5/1(CANMessage)
  [MCPInitialized] -> CAN TX5/2(MCPInitialized)
  CAN Rx/9(ID) -> CAN Pack4/1
  CAN Rx/10(Length) -> CAN Pack4/2
  Bus Selector16/2 -> Vector Concatenate1/1  "<Length>"
  Vector Concatenate3/1 -> MATLAB Function2/3(Data)
  Bus Selector16/1 -> Vector Concatenate/1  "<ID>"
  SPI Controller Transfer4/1 -> Terminator1/1
  MATLAB Function2/1(WriteInstruction) -> Vector Concatenate2/1
  Period/1 -> MATLAB Function2/5(period)
  Vector Concatenate2/1 -> SPI Controller Transfer4/1
  Bus Selector1/3 -> Vector Concatenate3/2  "<Data>"
  Bus Selector2/3 -> Vector Concatenate3/3  "<Data>"
  Bus Selector2/1 -> Vector Concatenate/3  "<ID>"
  TXBuffer/1 -> Vector Concatenate2/2
  Bus Selector16/3 -> Vector Concatenate3/1  "<Data>"
  RTS/1 -> MATLAB Function2/4(RTS)
  MATLAB Function2/2(CANVector) -> Vector Concatenate2/3
  Offset/1 -> MATLAB Function2/6(offset)
  Bus Selector1/1 -> Vector Concatenate/2  "<ID>"
  Vector Concatenate1/1 -> MATLAB Function2/2(Length)
  MATLAB Function2/3(RTSByte) -> SPI Controller Transfer5/1
  Bus Selector2/2 -> Vector Concatenate1/3  "<Length>"
  SPI Controller Transfer5/1 -> Terminator2/1
  Bus Selector1/2 -> Vector Concatenate1/2  "<Length>"
  Vector Concatenate/1 -> MATLAB Function2/1(ID)
  [MCPInitialized] -> CAN TX6/4(MCPInitialized)

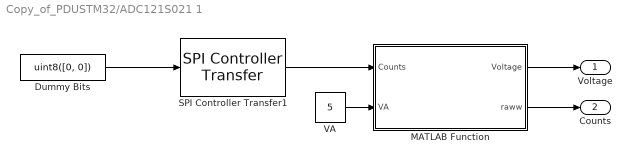
== system Copy_of_PDUSTM32/ADC121S021 1 ==
  Dummy Bits : Constant  Value=uint8([0, 0])
  MATLAB Function : MATLAB Function  TreatAsAtomicUnit=on
  SPI Controller Transfer1 : stm32blockslib/SPI Controller Transfer  Priority=2  SPIModuleSelect=SPI1  ClockPolarity=Low  ClockPhase=1 Edge  SPIModule=uint32(0)  Mode=Master  BusSpeed=uint32(1000000)  FirstBitToTransfer=Most significant bit (MSB)  ClockMode=0  BlockFunction=Transfer  EnableRegisterAddress=off  RegisterAddress=0  OutputDataType=uint8  OutputDataLength=1  OutputStatus=off  BlockingMode=on  Timeout=0.01  DataBits=8  UseCustomSSPin=Explicit GPIO calls  ActiveLowSSPin=Active low  Port_Select=GPIOA  Pin=0
      settings: LibrarySourceBlock=stm32h7xxblockslib/SPI Controller Transfer
  VA : Constant  Value=5  OutDataTypeStr=double
  Voltage : Outport  OutDataTypeStr=double
  Counts : Outport  Port=2  OutDataTypeStr=uint8
  wires:
  Dummy Bits/1 -> SPI Controller Transfer1/1
  SPI Controller Transfer1/1 -> MATLAB Function/1(Counts)
  VA/1 -> MATLAB Function/2(VA)
  MATLAB Function/1(Voltage) -> Voltage/1
  MATLAB Function/2(raww) -> Counts/1

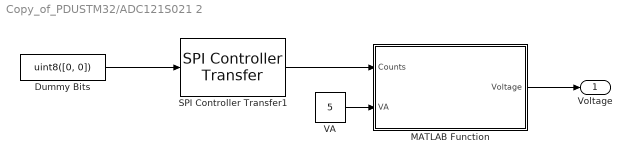
== system Copy_of_PDUSTM32/ADC121S021 2 ==
  Dummy Bits : Constant  Value=uint8([0, 0])
  MATLAB Function : MATLAB Function  TreatAsAtomicUnit=on
  SPI Controller Transfer1 : stm32blockslib/SPI Controller Transfer  Priority=2  SPIModuleSelect=SPI1  ClockPolarity=Low  ClockPhase=1 Edge  SPIModule=uint32(0)  Mode=Master  BusSpeed=uint32(1000000)  FirstBitToTransfer=Most significant bit (MSB)  ClockMode=0  BlockFunction=Transfer  EnableRegisterAddress=off  RegisterAddress=0  OutputDataType=uint8  OutputDataLength=1  OutputStatus=off  BlockingMode=on  Timeout=0.01  DataBits=8  UseCustomSSPin=Explicit GPIO calls  ActiveLowSSPin=Active low  Port_Select=GPIOA  Pin=1
      settings: LibrarySourceBlock=stm32h7xxblockslib/SPI Controller Transfer
  VA : Constant  Value=5
  Voltage : Outport  OutDataTypeStr=double
  wires:
  Dummy Bits/1 -> SPI Controller Transfer1/1
  SPI Controller Transfer1/1 -> MATLAB Function/1(Counts)
  VA/1 -> MATLAB Function/2(VA)
  MATLAB Function/1(Voltage) -> Voltage/1

== system Copy_of_PDUSTM32/ADC121S021 3 ==
  Dummy Bits : Constant  Value=uint8([0, 0])
  MATLAB Function : MATLAB Function  TreatAsAtomicUnit=on
  SPI Controller Transfer1 : stm32blockslib/SPI Controller Transfer  Priority=2  SPIModuleSelect=SPI1  ClockPolarity=Low  ClockPhase=1 Edge  SPIModule=uint32(0)  Mode=Master  BusSpeed=uint32(1000000)  FirstBitToTransfer=Most significant bit (MSB)  ClockMode=0  BlockFunction=Transfer  EnableRegisterAddress=off  RegisterAddress=0  OutputDataType=uint8  OutputDataLength=1  OutputStatus=off  BlockingMode=on  Timeout=0.01  DataBits=8  UseCustomSSPin=Explicit GPIO calls  ActiveLowSSPin=Active low  Port_Select=GPIOA  Pin=2
      settings: LibrarySourceBlock=stm32h7xxblockslib/SPI Controller Transfer
  VA : Constant  Value=5
  Voltage : Outport  OutDataTypeStr=double
  wires:
  Dummy Bits/1 -> SPI Controller Transfer1/1
  SPI Controller Transfer1/1 -> MATLAB Function/1(Counts)
  VA/1 -> MATLAB Function/2(VA)
  MATLAB Function/1(Voltage) -> Voltage/1

== system Copy_of_PDUSTM32/ADC121S021 4 ==
  Dummy Bits : Constant  Value=uint8([0, 0])
  MATLAB Function : MATLAB Function  TreatAsAtomicUnit=on
  SPI Controller Transfer1 : stm32blockslib/SPI Controller Transfer  Priority=2  SPIModuleSelect=SPI1  ClockPolarity=Low  ClockPhase=1 Edge  SPIModule=uint32(0)  Mode=Master  BusSpeed=uint32(1000000)  FirstBitToTransfer=Most significant bit (MSB)  ClockMode=0  BlockFunction=Transfer  EnableRegisterAddress=off  RegisterAddress=0  OutputDataType=uint8  OutputDataLength=1  OutputStatus=off  BlockingMode=on  Timeout=0.01  DataBits=8  UseCustomSSPin=Explicit GPIO calls  ActiveLowSSPin=Active low  Port_Select=GPIOB  Pin=10
      settings: LibrarySourceBlock=stm32h7xxblockslib/SPI Controller Transfer
  VA : Constant  Value=5
  Voltage : Outport  OutDataTypeStr=double
  wires:
  Dummy Bits/1 -> SPI Controller Transfer1/1
  SPI Controller Transfer1/1 -> MATLAB Function/1(Counts)
  VA/1 -> MATLAB Function/2(VA)
  MATLAB Function/1(Voltage) -> Voltage/1
